simulink model "rtwdemo_autosar_preprocessing"  (Simulink 7.6)
settings: Solver=FixedStepDiscrete  StartTime=0.0  StopTime=10.0  FixedStep=0.001  RelTol=1e-3
PreLoadFcn:
  | load rtwdemo_autosar_preprocessing_data.mat
settings Model: Creator=The MathWorks Inc.
settings DataIOCC: SaveFormat=StructureWithTime
settings OptimizationCC: InlineParams=on  ZeroExternalMemoryAtStartup=off  ZeroInternalMemoryAtStartup=off  OptimizeModelRefInitCode=on  LifeSpan=1
settings DebuggingCC: StrictBusMsg=Warning
settings HardwareCC: ProdIntDivRoundTo=Zero  ProdEndianess=LittleEndian  ProdHWDeviceType=Generic->32-bit Embedded Processor
settings SFSimCC: SimCustomHeaderCode="#include \"Rte_Type.h\""  SimUserIncludeDirs=$matlabroot$\toolbox\rtw\rtwdemos\autosartgt_demo  SimParseCustomCode=off
settings RTWCC: SystemTargetFile=autosar.tlc  GenCodeOnly=on  TemplateMakefile=ert_default_tmf  Description=AUTOSAR  GenerateReport=on  RTWVerbose=off  ProcessScript=autosar_make_rtw_hook  IncludeHyperlinkInReport=on  GenerateCodeInfo=on
settings CodeAppCC: IgnoreCustomStorageClasses=off
settings STFCustomTargetCC: CompOptLevelCompliant=on  IncludeMdlTerminateFcn=off  CombineOutputUpdateFcns=on  SuppressErrorStatus=on  ERTCustomFileBanners=on  SupportNonFinite=off  SupportComplex=off  SupportContinuousTime=off  SupportNonInlinedSFcns=off  PortableWordSizes=on  CPPClassGenCompliant=on  AutosarCompliant=on  SystemTargetFile=autosar.tlc
settings ERTTargetCC: MultiwordLength=2048  ParMdlRefBuildCompliant=off  IncludeMdlTerminateFcn=off  SuppressErrorStatus=on  ERTFirstTimeCompliant=off  SupportNonFinite=off  SupportComplex=off  PortableWordSizes=on  ModelStepFunctionPrototypeControlCompliant=off  AutosarCompliant=on  ExtModeMexFile=noextcomm  InlinedParameterPlacement=NonHierarchical  ERTCustomFileTemplate=example_file_process.tlc  ConvertIfToSwitch=off
settings CustomProperty: DataType=RTWOptions_EnumType__toolbox_rtw_targets_AUTOSAR_AUTOSAR_autosar_1_1AutosarSchemaVersion  Value=3.1
settings EnumStrPairs: String=2.0

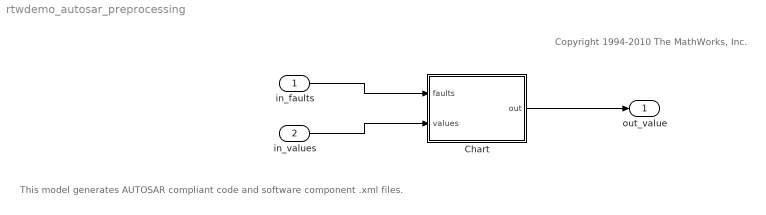
== system rtwdemo_autosar_preprocessing ==
  note: Copyright 1994-2010 The MathWorks, Inc.
  note: This model generates AUTOSAR compliant code and software component .xml files.
  in_faults : Inport  OutDataTypeStr=Bus: Boolean_pair  PortDimensions=1  BusOutputAsStruct=on
  in_values : Inport  Port=2  OutDataTypeStr=Bus: Double_pair  PortDimensions=1  BusOutputAsStruct=on
  Chart : Stateflow chart  TreatAsAtomicUnit=on
  out_value : Outport  OutMin=0.000000  OutMax=179769313486231570000000000000000000000000000000000000000000000000000000000000000000000000000000000000000000000000000000000000000000000000000000000000000000000000000000000000000000000000000000000000000000000000000000000000000000000000000000000000000000000000000000000000000000000000000000000000000000000000000.000000  OutDataTypeStr=double  PortDimensions=1
  wires:
  in_faults/1 -> Chart/1(faults)
  in_values/1 -> Chart/2(values)
  Chart/1(out) -> out_value/1

== stateflow chart Chart ==
  (default) -> (junction 3)
  (junction 3) -> (junction 4) [order 1] : [faults.primary == 0]{out = values.primary;}
  (junction 3) -> (junction 5) [order 2]
  (junction 5) -> (junction 6) [order 1] : [faults.secondary == 0]{out = values.secondary;}
  (junction 7) -> (junction 8) : {out = 1.0;}
  (junction 5) -> (junction 7) [order 2]
  data: faults input double; values input double; out output double
